simulink model "Week1_Q7"  (R2020b)
settings: Solver=VariableStepAuto  StartTime=0.0  StopTime=10.0  RelTol=1e-3
settings Model: Creator=DELL  LastModifiedBy=DELL

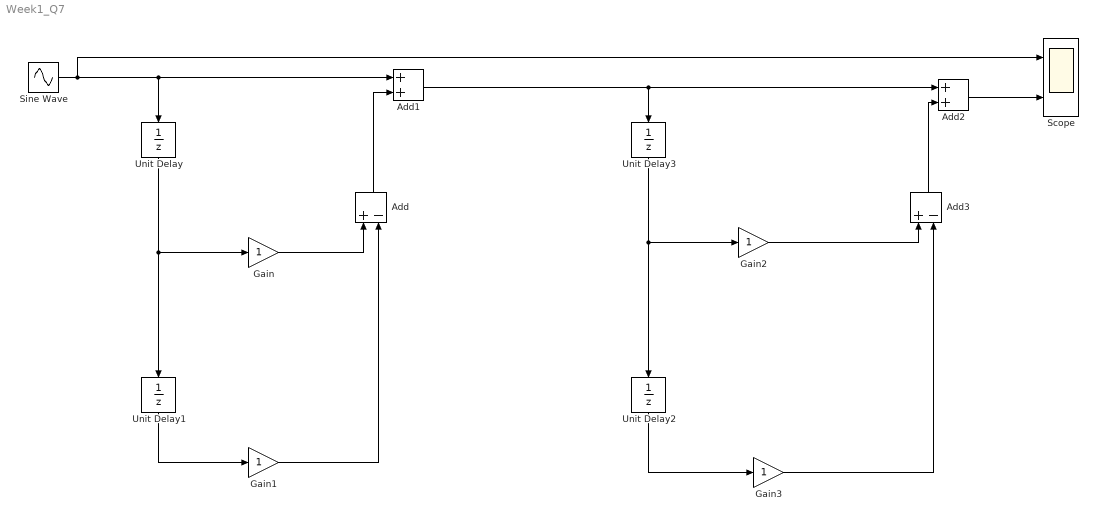
== system Week1_Q7 ==
  Add : Sum  Inputs=+-
  Add1 : Sum
  Add2 : Sum
  Add3 : Sum  Inputs=+-
  Gain{,1..3} (4 alike) : Gain
  Scope : Scope  NumInputPorts=2
  Sine Wave : Sin  SampleTime=0
  Unit Delay{,1..3} (4 alike) : UnitDelay  SampleTime=-1  HasFrameUpgradeWarning=on
  wires:
  Sine Wave/1 -> Scope/1, Unit Delay/1, Add1/1
  Unit Delay/1 -> Unit Delay1/1, Gain/1
  Gain/1 -> Add/1
  Add/1 -> Add1/2
  Unit Delay1/1 -> Gain1/1
  Gain1/1 -> Add/2
  Add1/1 -> Unit Delay3/1, Add2/1
  Unit Delay3/1 -> Unit Delay2/1, Gain2/1
  Gain2/1 -> Add3/1
  Unit Delay2/1 -> Gain3/1
  Gain3/1 -> Add3/2
  Add3/1 -> Add2/2
  Add2/1 -> Scope/2
